simulink model "SolveCurveAndPhasePlaneofDifferentialEquation"  (R2019b)
settings: Solver=VariableStepAuto  StartTime=0.0  StopTime=50  RelTol=1e-6  AbsTol=1e-5
libraries: simulink x1
settings Model: Creator=19398  LastModifiedBy=19398

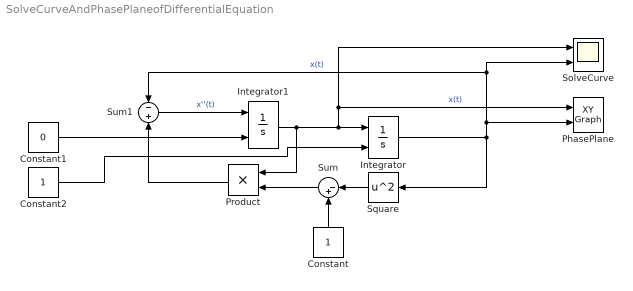
== system SolveCurveAndPhasePlaneofDifferentialEquation ==
  Constant : Constant
  Constant1 : Constant  Value=0
  Constant2 : Constant
  Integrator : Integrator  InitialConditionSource=external  InitialCondition=1
  Integrator1 : Integrator  InitialConditionSource=external
  PhasePlane : simulink/Sinks/XY Graph  xmin=-3  xmax=3  ymin=-3  ymax=3  st=-1
  Product : Product
  SolveCurve : Scope  NumInputPorts=2
  Square : Math  Operator=square  SignedPower=off  SaturateOnIntegerOverflow=on
  Sum : Sum  Inputs=|-+
  Sum1 : Sum  Inputs=-|+
  wires:
  Integrator1/1 -> Product/1, PhasePlane/1, SolveCurve/1, Integrator/1  "x(t)"
  Integrator/1 -> Square/1, PhasePlane/2, SolveCurve/2, Sum1/1  "x(t)"
  Square/1 -> Sum/1
  Constant/1 -> Sum/2
  Sum/1 -> Product/2
  Sum1/1 -> Integrator1/1  "x''(t)"
  Product/1 -> Sum1/2
  Constant1/1 -> Integrator1/2
  Constant2/1 -> Integrator/2
